simulink model "MyFiltrEnery"  (R2021a)
settings: Solver=VariableStepAuto  StartTime=0.0  StopTime=10.0  RelTol=1e-3
libraries: dspspect3 x1
settings Model: Creator=Alex  LastModifiedBy=Alex

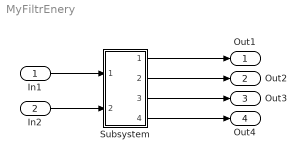
== system MyFiltrEnery ==
  In1 : Inport
  In2 : Inport  Port=2
  Subsystem : Subsystem
  Out1 : Outport
  Out2 : Outport  Port=2
  Out3 : Outport  Port=3
  Out4 : Outport  Port=4
  wires:
  In1/1 -> Subsystem/1(In1)
  In2/1 -> Subsystem/2(In2)
  Subsystem/1(Out1) -> Out1/1
  Subsystem/2(Out2) -> Out2/1
  Subsystem/3(Out3) -> Out3/1
  Subsystem/4(Out4) -> Out4/1

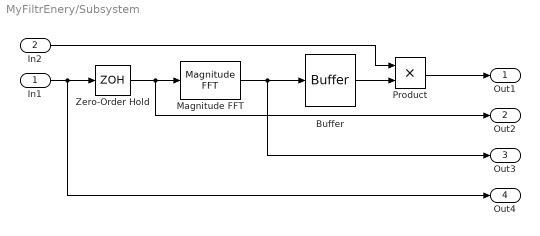
== system MyFiltrEnery/Subsystem ==
  In1 : Inport
  In2 : Inport  Port=2
  Buffer : Buffer  OutputFrames=off
  Magnitude FFT : dspspect3/Magnitude FFT  mag_or_magsq=Magnitude squared  FFTImplementation=Auto  fftLenInherit=off  fftsize=64  WrapInput=on
      settings: SourceProductBaseCode=DS
  Product : Product
  Zero-Order Hold : ZeroOrderHold  SampleTime=0.01
  Out1 : Outport
  Out2 : Outport  Port=2
  Out3 : Outport  Port=3
  Out4 : Outport  Port=4
  wires:
  Zero-Order Hold/1 -> Out2/1, Magnitude FFT/1
  In1/1 -> Out4/1, Zero-Order Hold/1
  Magnitude FFT/1 -> Out3/1, Buffer/1
  Buffer/1 -> Product/2
  Product/1 -> Out1/1
  In2/1 -> Product/1
